simulink library "ESSLibrary"  (R2020a)
settings: Solver=VariableStepAuto  StartTime=0.0  StopTime=10.0  RelTol=1e-3
libraries: $bdroot x82, powerlib_meascontrol x10, simulink x7
(part 2 of 7)

== system ESSLibrary/PostProcessing ==
  Enable : Inport  OutDataTypeStr=boolean
  ECPAppPow : Inport  Port=2  OutDataTypeStr=double
  ActivePowerPU : Inport  Port=3  OutDataTypeStr=double
  ReactivePowerPU : Inport  Port=4  OutDataTypeStr=double
  ElseActionSubsystem : Subsystem  TreatAsAtomicUnit=on
  If : If  IfExpression=u1 ~= 0
  If Action Subsystem : Subsystem  TreatAsAtomicUnit=on
  Switch1 : Switch  Criteria=u2 > Threshold
  Switch28 : Switch  Criteria=u2 > Threshold
  ActivePowerOut : Outport
  ReactivePowerOut : Outport  Port=2
  wires:
  If/1 -> If Action Subsystem/Action
  If/2 -> ElseActionSubsystem/Action
  Enable/1 -> Switch28/2, Switch1/2, If/1
  ActivePowerPU/1 -> If Action Subsystem/2(ActivePowerPU)
  [ElseActivePowerOut] -> Switch28/3
  ECPAppPow/1 -> If Action Subsystem/1(ECPAppPow)
  ReactivePowerPU/1 -> If Action Subsystem/3(ReactivePowerPU)
  If Action Subsystem/2(ReactivePowerOut) -> [IfReactivePowerOut]
  If Action Subsystem/1(ActivePowerOut) -> [IfActivePowerOut]
  [IfActivePowerOut] -> Switch28/1
  [IfReactivePowerOut] -> Switch1/1
  [ElseReactivePowerOut] -> Switch1/3
  Switch28/1 -> ActivePowerOut/1
  Switch1/1 -> ReactivePowerOut/1
  ElseActionSubsystem/1(ActivePowerOut) -> [ElseActivePowerOut]
  ElseActionSubsystem/2(ReactivePowerOut) -> [ElseReactivePowerOut]

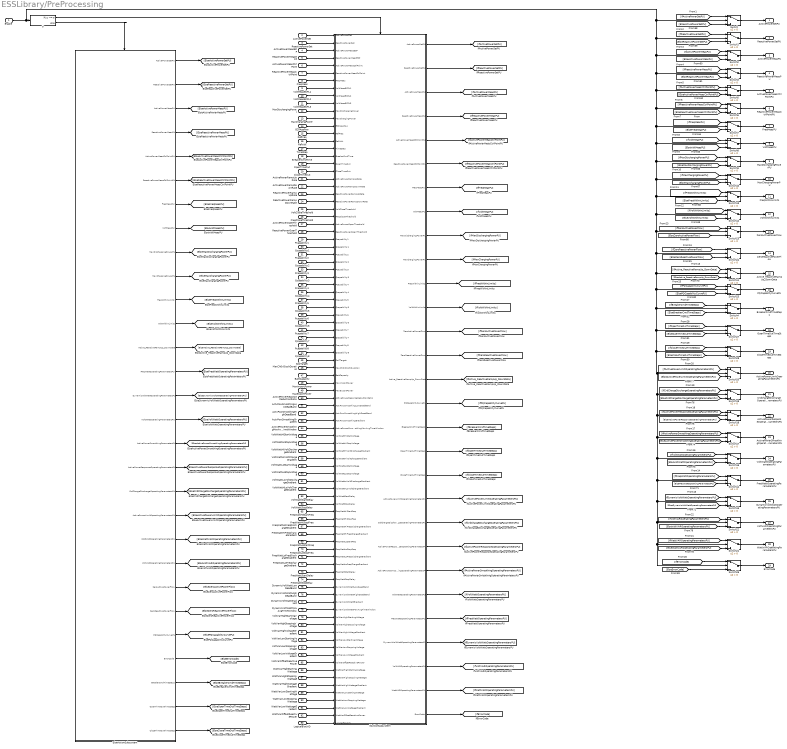
== system ESSLibrary/PreProcessing ==
  Enable : Inport  OutDataTypeStr=boolean
  ActivePowerSet : Inport  Port=2  OutDataTypeStr=double
  "ReactivePowerSet " : Inport  Port=3  OutDataTypeStr=double
  ActivePowerMeasECP : Inport  Port=4  OutDataTypeStr=double
  ReactivePowerMeasECP : Inport  Port=5  OutDataTypeStr=double
  ActivePowerMeasCtrlPoint : Inport  Port=6  OutDataTypeStr=double
  ReactivePowerMeasCtrlPoint : Inport  Port=7  OutDataTypeStr=double
  FreqMeas : Inport  Port=8  OutDataTypeStr=double
  VoltMeasECPL1 : Inport  Port=9  OutDataTypeStr=double
  VoltMeasECPL2 : Inport  Port=10  OutDataTypeStr=double
  VoltMeasECPL3 : Inport  Port=11  OutDataTypeStr=double
  MaxDischargingPower : Inport  Port=12  OutDataTypeStr=double
  MaxChargingPower : Inport  Port=13  OutDataTypeStr=double
  ECPAppPow : Inport  Port=14  OutDataTypeStr=double
  RefFreq : Inport  Port=15  OutDataTypeStr=double
  RefVolt : Inport  Port=16  OutDataTypeStr=double
  TimeStep : Inport  Port=17  OutDataTypeStr=double
  BreakerCmdTime : Inport  Port=18  OutDataTypeStr=double
  OpenTimeOut : Inport  Port=19  OutDataTypeStr=double
  CloseTimeOut : Inport  Port=20  OutDataTypeStr=double
  ActivePowerRampUpRate : Inport  Port=21  OutDataTypeStr=double
  ActivePowerRampDownRate : Inport  Port=22  OutDataTypeStr=double
  ReactivePowerRampUpRate : Inport  Port=23  OutDataTypeStr=double
  ReactivePowerRampDownRate : Inport  Port=24  OutDataTypeStr=double
  VoltCloseThreshold : Inport  Port=25  OutDataTypeStr=double
  FreqCloseThreshold : Inport  Port=26  OutDataTypeStr=double
  ActivePowerOpenThreshold : Inport  Port=27  OutDataTypeStr=double
  ReactivePowerOpenThreshold : Inport  Port=28  OutDataTypeStr=double
  Pcapability1 : Inport  Port=29  OutDataTypeStr=double
  Qcapability1 : Inport  Port=30  OutDataTypeStr=double
  Pcapability2 : Inport  Port=31  OutDataTypeStr=double
  Qcapability2 : Inport  Port=32  OutDataTypeStr=double
  Pcapability3 : Inport  Port=33  OutDataTypeStr=double
  Qcapability3 : Inport  Port=34  OutDataTypeStr=double
  Pcapability4 : Inport  Port=35  OutDataTypeStr=double
  Qcapability4 : Inport  Port=36  OutDataTypeStr=double
  Pcapability5 : Inport  Port=37  OutDataTypeStr=double
  Qcapability5 : Inport  Port=38  OutDataTypeStr=double
  Pcapability6 : Inport  Port=39  OutDataTypeStr=double
  Qcapability6 : Inport  Port=40  OutDataTypeStr=double
  Pcapability7 : Inport  Port=41  OutDataTypeStr=double
  Qcapability7 : Inport  Port=42  OutDataTypeStr=double
  Pcapability8 : Inport  Port=43  OutDataTypeStr=double
  Qcapability8 : Inport  Port=44  OutDataTypeStr=double
  SoCTarget : Inport  Port=45  OutDataTypeStr=double
  MaxChOrDischDuration : Inport  Port=46  OutDataTypeStr=double
  BattCapacity : Inport  Port=47  OutDataTypeStr=double
  MaxImportPower : Inport  Port=48  OutDataTypeStr=double
  MaxExportPower : Inport  Port=49  OutDataTypeStr=double
  ActivePowerReponseReductionRatio : Inport  Port=50  OutDataTypeStr=double
  ActvPowSmoothingLowDeadBand : Inport  Port=51  OutDataTypeStr=double
  ActvPowSmoothingHighDeadBand : Inport  Port=52  OutDataTypeStr=double
  ActvPowSmoothingGradient : Inport  Port=53  OutDataTypeStr=double
  ActivePowerSmoothingMovAvgTimeWindow : Inport  Port=54  OutDataTypeStr=double
  VoltWattHiStartVoltage : Inport  Port=55  OutDataTypeStr=double
  VoltWattHiStopVoltage : Inport  Port=56  OutDataTypeStr=double
  VoltWattHiVoltDischargeGradient : Inport  Port=57  OutDataTypeStr=double
  VoltWattHiVoltChargeGradient : Inport  Port=58  OutDataTypeStr=double
  VoltWattLoStartVoltage : Inport  Port=59  OutDataTypeStr=double
  VoltWattLoStopVoltage : Inport  Port=60  OutDataTypeStr=double
  VoltWattLoVoltDischargeGradient : Inport  Port=61  OutDataTypeStr=double
  VoltWattHLoVoltChargeGradient : Inport  Port=62  OutDataTypeStr=double
  VoltWattStartDelay : Inport  Port=63  OutDataTypeStr=double
  VoltWattStopDelay : Inport  Port=64  OutDataTypeStr=double
  FreqWattHiStartFreq : Inport  Port=65  OutDataTypeStr=double
  FreqWattHiStopFreq : Inport  Port=66  OutDataTypeStr=double
  FreqWattHiFreqDischargeGradient : Inport  Port=67  OutDataTypeStr=double
  FreqWattHiFreqChargeGradient : Inport  Port=68  OutDataTypeStr=double
  FreqWattLoStartFreq : Inport  Port=69  OutDataTypeStr=double
  FreqWattLoStopFreq : Inport  Port=70  OutDataTypeStr=double
  FreqWattLoFreqDischargeGradient : Inport  Port=71  OutDataTypeStr=double
  FreqWattLoFreqChargeGradient : Inport  Port=72  OutDataTypeStr=double
  FreqWattStartDelay : Inport  Port=73  OutDataTypeStr=double
  FreqWattStopDelay : Inport  Port=74  OutDataTypeStr=double
  DynamicVoltWattLowDeadBand : Inport  Port=75  OutDataTypeStr=double
  DynamicVoltWattHighDeadBand : Inport  Port=76  OutDataTypeStr=double
  DynamicVoltWattGradient : Inport  Port=77  OutDataTypeStr=double
  DynamicVoltWattMovAvgTimeWindow : Inport  Port=78  OutDataTypeStr=double
  VoltVarHighStartingVoltage : Inport  Port=79  OutDataTypeStr=double
  VoltVarHighStoppingVoltage : Inport  Port=80  OutDataTypeStr=double
  VoltVarHighVoltageGradient : Inport  Port=81  OutDataTypeStr=double
  VoltVarLowStartingVoltage : Inport  Port=82  OutDataTypeStr=double
  VoltVarLowStoppingVoltage : Inport  Port=83  OutDataTypeStr=double
  VoltVarLowVoltageGradient : Inport  Port=84  OutDataTypeStr=double
  VoltVarOffsetReactivePower : Inport  Port=85  OutDataTypeStr=double
  WattVarHighStartingWattage : Inport  Port=86  OutDataTypeStr=double
  WattVarHighStoppingWattage : Inport  Port=87  OutDataTypeStr=double
  WattVarHighWattageGradient : Inport  Port=88  OutDataTypeStr=double
  WattVarLowStartingWattage : Inport  Port=89  OutDataTypeStr=double
  WattVarLowStoppingWattage : Inport  Port=90  OutDataTypeStr=double
  WattVarLowWattageGradient : Inport  Port=91  OutDataTypeStr=double
  WattVarOffsetReactivePower : Inport  Port=92  OutDataTypeStr=double
  LogicalBlockID : Inport  Port=93  OutDataTypeStr=int32
  ElseActionSubsystem : Subsystem  TreatAsAtomicUnit=on
  If : If  IfExpression=u1 ~= 0
  IfActionSubsystem : Subsystem  TreatAsAtomicUnit=on
  Switch : Switch  Criteria=u2 > Threshold
  Switch{1..25,27..28} (27 alike) : Switch  Criteria=u2 > Threshold  OutDataTypeStr=Inherit: Inherit via back propagation
  Switch26 : Switch  Criteria=u2 > Threshold
  ActivePowerSetPU : Outport  OutDataTypeStr=double
  "ReactivePowerSetPU " : Outport  Port=2  OutDataTypeStr=double
  ActivePowerMeasPU : Outport  Port=3  OutDataTypeStr=double
  ReactivePowerMeasPU : Outport  Port=4  OutDataTypeStr=double
  ActivePowerMeasCtrlPointPU : Outport  Port=5  OutDataTypeStr=double
  ReactivePowerMeasCtrlPointPU : Outport  Port=6  OutDataTypeStr=double
  FreqMeasPU : Outport  Port=7  OutDataTypeStr=double
  VoltMeasPU : Outport  Port=8  OutDataTypeStr=double
  MaxDischargingPowerPU : Outport  Port=9  OutDataTypeStr=double
  MaxChargingPowerPU : Outport  Port=10  OutDataTypeStr=double
  FreqWithinLimits : Outport  Port=11  OutDataTypeStr=boolean
  VoltWithinLimits : Outport  Port=12  OutDataTypeStr=boolean
  ZeroActivePowerFlow : Outport  Port=13  OutDataTypeStr=boolean
  ZeroReactivePowerFlow : Outport  Port=14  OutDataTypeStr=boolean
  Active_ReactiveRampUp_DownData : Outport  Port=15  OutDataTypeStr=Bus: Active_ReactiveRampUp_DownData
  PQCapabiltyCurvePU : Outport  Port=16  OutDataTypeStr=double
  BreakerCmdTimeSteps : Outport  Port=17  OutDataTypeStr=int16
  OpenTimeOutTimeSteps : Outport  Port=18  OutDataTypeStr=int16
  CloseTimeOutTimeSteps : Outport  Port=19  OutDataTypeStr=int16
  ActivePowerLimitOperatingParametersPU : Outport  Port=20  OutDataTypeStr=Bus: ActivePowerLimitOperatingParametersPU
  CrdChargeDischargeOperatingParametersPU : Outport  Port=21
  ActivePowerResponseOperatingParametersPU : Outport  Port=22  OutDataTypeStr=Bus: ActivePowerResponseOperatingParametersPU
  ActivePowerSmoothingOperatingParametersPU : Outport  Port=23  OutDataTypeStr=Bus: ActivePowerSmoothingOperatingParametersPU
  VoltWattOperatingParametersPU : Outport  Port=24  OutDataTypeStr=Bus: VoltWattOperatingParametersPU
  FreqWattOperatingParametersPU : Outport  Port=25  OutDataTypeStr=Bus: FreqWattOperatingParametersPU
  DynamicVoltWattOperatingParametersPU : Outport  Port=26  OutDataTypeStr=Bus: DynamicVoltWattOperatingParameters
  VoltVAROperatingParametersPU : Outport  Port=27  OutDataTypeStr=Bus: VoltVarOperatingParametersPU
  WattVAROperatingParametersPU : Outport  Port=28  OutDataTypeStr=Bus: WattVarOperatingParametersPU
  ErrorCode : Outport  Port=29  OutDataTypeStr=uint32
  wires:
  If/1 -> IfActionSubsystem/Action
  If/2 -> ElseActionSubsystem/Action
  ActivePowerSet/1 -> IfActionSubsystem/1(ActivePowerSet)
  MaxDischargingPower/1 -> IfActionSubsystem/11(MaxDischargingPower)
  MaxChargingPower/1 -> IfActionSubsystem/12(MaxChargingPower)
  "ReactivePowerSet "/1 -> IfActionSubsystem/2("ReactivePowerSet ")
  ActivePowerMeasECP/1 -> IfActionSubsystem/3(ActivePowerMeasECP)
  ReactivePowerMeasECP/1 -> IfActionSubsystem/4(ReactivePowerMeasECP)
  ActivePowerMeasCtrlPoint/1 -> IfActionSubsystem/5(ActivePowerMeasCtrlPoint)
  ReactivePowerMeasCtrlPoint/1 -> IfActionSubsystem/6(ReactivePowerMeasCtrlPoint)
  ActivePowerOpenThreshold/1 -> IfActionSubsystem/26(ActivePowerOpenThreshold)
  FreqMeas/1 -> IfActionSubsystem/7(FreqMeas)
  FreqCloseThreshold/1 -> IfActionSubsystem/25(FreqCloseThreshold)
  VoltMeasECPL1/1 -> IfActionSubsystem/8(VoltMeasECPL1)
  VoltMeasECPL2/1 -> IfActionSubsystem/9(VoltMeasECPL2)
  VoltMeasECPL3/1 -> IfActionSubsystem/10(VoltMeasECPL3)
  RefVolt/1 -> IfActionSubsystem/15(RefVolt)
  RefFreq/1 -> IfActionSubsystem/14(RefFreq)
  ECPAppPow/1 -> IfActionSubsystem/13(ECPAppPow)
  VoltCloseThreshold/1 -> IfActionSubsystem/24(VoltCloseThreshold)
  ReactivePowerOpenThreshold/1 -> IfActionSubsystem/27(ReactivePowerOpenThreshold)
  IfActionSubsystem/29(ErrorCode) -> [IfErrorCode]
  IfActionSubsystem/8(VoltMeasPU) -> [IfVoltMeasPU]
  IfActionSubsystem/7(FreqMeasPU) -> [IfFreqMeasPU]
  IfActionSubsystem/6(ReactivePowerMeasCtrlPointPU) -> [IfReactivePowerMeasCtrlPointPU]
  IfActionSubsystem/5(ActivePowerMeasCtrlPointPU) -> [IfActivePowerMeasCtrlPointPU]
  IfActionSubsystem/4(ReactivePowerMeasPU) -> [IfReactivePowerMeasPU]
  IfActionSubsystem/2("ReactivePowerSetPU ") -> [IfReactivePowerSetPU]
  IfActionSubsystem/3(ActivePowerMeasPU) -> [IfActivePowerMeasPU]
  IfActionSubsystem/1(ActivePowerSetPU) -> [IfActivePowerSetPU]
  IfActionSubsystem/9(MaxDischargingPowerPU) -> [IfMaxDischargingPowerPU]
  IfActionSubsystem/10(MaxChargingPowerPU) -> [IfMaxChargingPowerPU]
  Switch/1 -> ActivePowerSetPU/1
  Switch1/1 -> "ReactivePowerSetPU "/1
  Switch2/1 -> ActivePowerMeasPU/1
  Switch3/1 -> ReactivePowerMeasPU/1
  Switch5/1 -> ActivePowerMeasCtrlPointPU/1
  Switch6/1 -> ReactivePowerMeasCtrlPointPU/1
  Switch7/1 -> FreqMeasPU/1
  Switch8/1 -> VoltMeasPU/1
  Switch9/1 -> MaxDischargingPowerPU/1
  Switch10/1 -> MaxChargingPowerPU/1
  IfActionSubsystem/11(FreqWithinLimits) -> [IfFreqWithinLimits]
  IfActionSubsystem/12(VoltWithinLimits) -> [IfVoltWithinLimits]
  Switch12/1 -> VoltWithinLimits/1
  Switch13/1 -> FreqWithinLimits/1
  Enable/1 -> Switch/2, Switch1/2, Switch2/2, Switch3/2, Switch5/2, Switch6/2, Switch7/2, Switch8/2, Switch9/2, Switch10/2, Switch13/2, Switch12/2, Switch23/2, Switch11/2, Switch4/2, Switch28/2, Switch20/2, Switch26/2, Switch21/2, Switch22/2, Switch15/2, Switch14/2, Switch16/2, Switch17/2, Switch18/2, Switch19/2, Switch27/2, Switch25/2, Switch24/2, If/1
  ReactivePowerRampUpRate/1 -> IfActionSubsystem/22(ReactivePowerRampUpRate)
  ReactivePowerRampDownRate/1 -> IfActionSubsystem/23(ReactivePowerRampDownRate)
  ActivePowerRampDownRate/1 -> IfActionSubsystem/21(ActivePowerRampDownRate)
  ActivePowerRampUpRate/1 -> IfActionSubsystem/20(ActivePowerRampUpRate)
  TimeStep/1 -> IfActionSubsystem/16(TimeStep)
  MaxImportPower/1 -> IfActionSubsystem/47(MaxImportPower)
  WattVarLowStartingWattage/1 -> IfActionSubsystem/88(WattVarLowStartingWattage)
  WattVarHighWattageGradient/1 -> IfActionSubsystem/87(WattVarHighWattageGradient)
  FreqWattHiStartFreq/1 -> IfActionSubsystem/64(FreqWattHiStartFreq)
  FreqWattHiStopFreq/1 -> IfActionSubsystem/65(FreqWattHiStopFreq)
  FreqWattHiFreqDischargeGradient/1 -> IfActionSubsystem/66(FreqWattHiFreqDischargeGradient)
  FreqWattHiFreqChargeGradient/1 -> IfActionSubsystem/67(FreqWattHiFreqChargeGradient)
  FreqWattLoStopFreq/1 -> IfActionSubsystem/69(FreqWattLoStopFreq)
  FreqWattLoStartFreq/1 -> IfActionSubsystem/68(FreqWattLoStartFreq)
  FreqWattLoFreqDischargeGradient/1 -> IfActionSubsystem/70(FreqWattLoFreqDischargeGradient)
  FreqWattLoFreqChargeGradient/1 -> IfActionSubsystem/71(FreqWattLoFreqChargeGradient)
  DynamicVoltWattHighDeadBand/1 -> IfActionSubsystem/75(DynamicVoltWattHighDeadBand)
  DynamicVoltWattLowDeadBand/1 -> IfActionSubsystem/74(DynamicVoltWattLowDeadBand)
  DynamicVoltWattGradient/1 -> IfActionSubsystem/76(DynamicVoltWattGradient)
  DynamicVoltWattMovAvgTimeWindow/1 -> IfActionSubsystem/77(DynamicVoltWattMovAvgTimeWindow)
  VoltWattHiStartVoltage/1 -> IfActionSubsystem/54(VoltWattHiStartVoltage)
  VoltWattHiStopVoltage/1 -> IfActionSubsystem/55(VoltWattHiStopVoltage)
  VoltWattHiVoltDischargeGradient/1 -> IfActionSubsystem/56(VoltWattHiVoltDischargeGradient)
  VoltWattHiVoltChargeGradient/1 -> IfActionSubsystem/57(VoltWattHiVoltChargeGradient)
  ActvPowSmoothingLowDeadBand/1 -> IfActionSubsystem/50(ActvPowSmoothingLowDeadBand)
  ActvPowSmoothingHighDeadBand/1 -> IfActionSubsystem/51(ActvPowSmoothingHighDeadBand)
  ActivePowerSmoothingMovAvgTimeWindow/1 -> IfActionSubsystem/53(ActivePowerSmoothingMovAvgTimeWindow)
  ActivePowerReponseReductionRatio/1 -> IfActionSubsystem/49(ActivePowerReponseReductionRatio)
  SoCTarget/1 -> IfActionSubsystem/44(SoCTarget)
  MaxChOrDischDuration/1 -> IfActionSubsystem/45(MaxChOrDischDuration)
  WattVarHighStartingWattage/1 -> IfActionSubsystem/85(WattVarHighStartingWattage)
  WattVarHighStoppingWattage/1 -> IfActionSubsystem/86(WattVarHighStoppingWattage)
  VoltVarHighStartingVoltage/1 -> IfActionSubsystem/78(VoltVarHighStartingVoltage)
  VoltVarHighStoppingVoltage/1 -> IfActionSubsystem/79(VoltVarHighStoppingVoltage)
  VoltVarHighVoltageGradient/1 -> IfActionSubsystem/80(VoltVarHighVoltageGradient)
  VoltVarLowStartingVoltage/1 -> IfActionSubsystem/81(VoltVarLowStartingVoltage)
  Pcapability1/1 -> IfActionSubsystem/28(Pcapability1)
  Qcapability1/1 -> IfActionSubsystem/29(Qcapability1)
  Pcapability2/1 -> IfActionSubsystem/30(Pcapability2)
  Qcapability2/1 -> IfActionSubsystem/31(Qcapability2)
  Pcapability3/1 -> IfActionSubsystem/32(Pcapability3)
  Qcapability3/1 -> IfActionSubsystem/33(Qcapability3)
  Pcapability4/1 -> IfActionSubsystem/34(Pcapability4)
  Qcapability4/1 -> IfActionSubsystem/35(Qcapability4)
  Pcapability5/1 -> IfActionSubsystem/36(Pcapability5)
  Qcapability5/1 -> IfActionSubsystem/37(Qcapability5)
  Pcapability6/1 -> IfActionSubsystem/38(Pcapability6)
  Qcapability6/1 -> IfActionSubsystem/39(Qcapability6)
  Pcapability7/1 -> IfActionSubsystem/40(Pcapability7)
  Qcapability7/1 -> IfActionSubsystem/41(Qcapability7)
  Pcapability8/1 -> IfActionSubsystem/42(Pcapability8)
  Qcapability8/1 -> IfActionSubsystem/43(Qcapability8)
  LogicalBlockID/1 -> IfActionSubsystem/92(LogicalBlockID)
  ActvPowSmoothingGradient/1 -> IfActionSubsystem/52(ActvPowSmoothingGradient)
  WattVarLowWattageGradient/1 -> IfActionSubsystem/90(WattVarLowWattageGradient)
  VoltVarOffsetReactivePower/1 -> IfActionSubsystem/84(VoltVarOffsetReactivePower)
  VoltVarLowVoltageGradient/1 -> IfActionSubsystem/83(VoltVarLowVoltageGradient)
  VoltVarLowStoppingVoltage/1 -> IfActionSubsystem/82(VoltVarLowStoppingVoltage)
  BattCapacity/1 -> IfActionSubsystem/46(BattCapacity)
  MaxExportPower/1 -> IfActionSubsystem/48(MaxExportPower)
  VoltWattLoStartVoltage/1 -> IfActionSubsystem/58(VoltWattLoStartVoltage)
  VoltWattLoStopVoltage/1 -> IfActionSubsystem/59(VoltWattLoStopVoltage)
  VoltWattLoVoltDischargeGradient/1 -> IfActionSubsystem/60(VoltWattLoVoltDischargeGradient)
  VoltWattHLoVoltChargeGradient/1 -> IfActionSubsystem/61(VoltWattHLoVoltChargeGradient)
  VoltWattStartDelay/1 -> IfActionSubsystem/62(VoltWattStartDelay)
  VoltWattStopDelay/1 -> IfActionSubsystem/63(VoltWattStopDelay)
  WattVarLowStoppingWattage/1 -> IfActionSubsystem/89(WattVarLowStoppingWattage)
  WattVarOffsetReactivePower/1 -> IfActionSubsystem/91(WattVarOffsetReactivePower)
  FreqWattStopDelay/1 -> IfActionSubsystem/73(FreqWattStopDelay)
  FreqWattStartDelay/1 -> IfActionSubsystem/72(FreqWattStartDelay)
  IfActionSubsystem/15(Active_ReactiveRampUp_DownData) -> [IfActive_ReactiveRampUp_DownData]
  IfActionSubsystem/25(FreqWattOperatingParametersPU) -> [IfFreqWattOperatingParametersPU]
  IfActionSubsystem/26(DynamicVoltWattOperatingParametersPU) -> [IfDynamicVoltWattOperatingParametersPU]
  IfActionSubsystem/24(VoltWattOperatingParametersPU) -> [IfVoltWattOperatingParametersPU]
  IfActionSubsystem/23(ActivePowerSmoothingOperatingParametersPU) -> [IfActivePowerSmoothingOperatingParametersPU]
  IfActionSubsystem/21(CrdChargeDischargeOperatingParametersPU) -> [IfCrdChargeDischargeOperatingParametersPU]
  IfActionSubsystem/20(ActivePowerLimitOperatingParametersPU) -> [IfActivePowerLimitOperatingParametersPU]
  IfActionSubsystem/28(WattVAROperatingParametersPU) -> [IfWattVAROperatingParametersPU]
  IfActionSubsystem/27(VoltVAROperatingParametersPU) -> [IfVoltVAROperatingParametersPU]
  IfActionSubsystem/13(ZeroActivePowerFlow) -> [IfZeroActivePowerFlow]
  IfActionSubsystem/14(ZeroReactivePowerFlow) -> [IfZeroReactivePowerFlow]
  IfActionSubsystem/16(PQCapabiltyCurvePU) -> [IfPQCapabilityCurvePU]
  ElseActionSubsystem/1(ActivePowerSetPU) -> [ElseActivePowerSetPU]
  ElseActionSubsystem/2("ReactivePowerSetPU ") -> [ElseReactivePowerSetPU]
  ElseActionSubsystem/3(ActivePowerMeasPU) -> [ElseActivePowerMeasPU]
  ElseActionSubsystem/4(ReactivePowerMeasPU) -> [ElseReactivePowerMeasPU]
  ElseActionSubsystem/5(ActivePowerMeasCtrlPointPU) -> [ElseActivePowerMeasCtrlPointPU]
  ElseActionSubsystem/6(ReactivePowerMeasCtrlPointPU) -> [ElseReactivePowerMeasCtrlPointPU]
  ElseActionSubsystem/7(FreqMeasPU) -> [ElseFreqMeasPU]
  ElseActionSubsystem/8(VoltMeasPU) -> [ElseVoltMeasPU]
  ElseActionSubsystem/9(MaxDischargingPowerPU) -> [ElseMaxDischargingPowerPU]
  ElseActionSubsystem/10(MaxChargingPowerPU) -> [ElseMaxChargingPowerPU]
  ElseActionSubsystem/11(FreqWithinLimits) -> [ElseFreqWithinLimits]
  ElseActionSubsystem/12(VoltWithinLimits) -> [ElseVoltWithinLimits]
  ElseActionSubsystem/13(Active_ReactiveRampUp_DownData) -> [ElseActive_ReactiveRampUp_DownData]
  ElseActionSubsystem/14(FreqWattOperatingParametersPU) -> [ElseFreqWattOperatingParametersPU]
  ElseActionSubsystem/15(DynamicVoltWattOperatingParametersPU) -> [ElseDynamicVoltWattOperatingParametersPU]
  ElseActionSubsystem/16(VoltWattOperatingParametersPU) -> [ElseVoltWattOperatingParametersPU]
  ElseActionSubsystem/17(ActivePowerSmoothingParametersPU) -> [ElseActivePowerSmoothingOperatingParametersPU]
  ElseActionSubsystem/18(ActivePowerResponseOperatingParametersPU) -> [ElseActivePowerResponseOperatingParametersPU]
  ElseActionSubsystem/19(CrdChargeDischargeOperatingParametersPU) -> [ElseCrdChargeDischargeOperatingParametersPU]
  ElseActionSubsystem/20(ActivePowerLimitOperatingParametersPU) -> [ElseActivePowerLimitOperatingParametersPU]
  ElseActionSubsystem/21(WattVAROperatingParametersPU) -> [ElseWattVAROperatingParametersPU]
  ElseActionSubsystem/22(VoltVAROperatingParametersPU) -> [ElseVoltVAROperatingParametersPU]
  ElseActionSubsystem/23(ZeroActivePowerFlow) -> [ElseZeroActivePowerFlow]
  ElseActionSubsystem/24(ZeroReactivePowerFlow) -> [ElseZeroReactivePowerFlow]
  ElseActionSubsystem/25(PQCapabiltyCurvePU) -> [ElsePQCapabilityCurvePU]
  ElseActionSubsystem/26(ErrorCode) -> [ElseErrorCode]
  [ElseActivePowerSetPU] -> Switch/3
  [ElseReactivePowerSetPU] -> Switch1/3
  [ElseActivePowerMeasPU] -> Switch2/3
  [ElseReactivePowerMeasPU] -> Switch3/3
  [ElseActivePowerMeasCtrlPointPU] -> Switch5/3
  [ElseReactivePowerMeasCtrlPointPU] -> Switch6/3
  [ElseFreqMeasPU] -> Switch7/3
  [ElseVoltMeasPU] -> Switch8/3
  [ElseMaxDischargingPowerPU] -> Switch9/3
  [ElseMaxChargingPowerPU] -> Switch10/3
  [ElseFreqWithinLimits] -> Switch13/3
  [ElseVoltWithinLimits] -> Switch12/3
  [ElseActive_ReactiveRampUp_DownData] -> Switch11/3
  [ElseFreqWattOperatingParametersPU] -> Switch14/3
  [ElseDynamicVoltWattOperatingParametersPU] -> Switch15/3
  [ElseVoltWattOperatingParametersPU] -> Switch16/3
  [ElseActivePowerSmoothingOperatingParametersPU] -> Switch17/3
  [ElseActivePowerResponseOperatingParametersPU] -> Switch18/3
  [ElseCrdChargeDischargeOperatingParametersPU] -> Switch19/3
  [ElseActivePowerLimitOperatingParametersPU] -> Switch20/3
  [ElseWattVAROperatingParametersPU] -> Switch21/3
  [ElseVoltVAROperatingParametersPU] -> Switch22/3
  [ElseZeroActivePowerFlow] -> Switch23/3
  [ElseZeroReactivePowerFlow] -> Switch24/3
  [ElsePQCapabilityCurvePU] -> Switch25/3
  [ElseErrorCode] -> Switch26/3
  [IfActivePowerSetPU] -> Switch/1
  [IfReactivePowerSetPU] -> Switch1/1
  [IfActivePowerMeasPU] -> Switch2/1
  [IfReactivePowerMeasPU] -> Switch3/1
  [IfActivePowerMeasCtrlPointPU] -> Switch5/1
  [IfReactivePowerMeasCtrlPointPU] -> Switch6/1
  [IfFreqMeasPU] -> Switch7/1
  [IfVoltMeasPU] -> Switch8/1
  [IfMaxDischargingPowerPU] -> Switch9/1
  [IfMaxChargingPowerPU] -> Switch10/1
  [IfFreqWithinLimits] -> Switch13/1
  [IfVoltWithinLimits] -> Switch12/1
  [IfActive_ReactiveRampUp_DownData] -> Switch11/1
  [IfFreqWattOperatingParametersPU] -> Switch14/1
  [IfDynamicVoltWattOperatingParametersPU] -> Switch15/1
  [IfVoltWattOperatingParametersPU] -> Switch16/1
  [IfActivePowerSmoothingOperatingParametersPU] -> Switch17/1
  [IfActivePowerResponseOperatingParametersPU] -> Switch18/1
  [IfCrdChargeDischargeOperatingParametersPU] -> Switch19/1
  [IfActivePowerLimitOperatingParametersPU] -> Switch20/1
  [IfWattVAROperatingParametersPU] -> Switch21/1
  [IfVoltVAROperatingParametersPU] -> Switch22/1
  [IfZeroActivePowerFlow] -> Switch23/1
  [IfZeroReactivePowerFlow] -> Switch24/1
  [IfPQCapabilityCurvePU] -> Switch25/1
  [IfErrorCode] -> Switch26/1
  IfActionSubsystem/22(ActivePowerResponseOperatingParametersPU) -> [IfActivePowerResponseOperatingParametersPU]
  Switch14/1 -> FreqWattOperatingParametersPU/1
  Switch15/1 -> DynamicVoltWattOperatingParametersPU/1
  Switch16/1 -> VoltWattOperatingParametersPU/1
  Switch17/1 -> ActivePowerSmoothingOperatingParametersPU/1
  Switch18/1 -> ActivePowerResponseOperatingParametersPU/1
  Switch19/1 -> CrdChargeDischargeOperatingParametersPU/1
  Switch20/1 -> ActivePowerLimitOperatingParametersPU/1
  Switch21/1 -> WattVAROperatingParametersPU/1
  Switch22/1 -> VoltVAROperatingParametersPU/1
  Switch23/1 -> ZeroActivePowerFlow/1
  Switch24/1 -> ZeroReactivePowerFlow/1
  Switch25/1 -> PQCapabiltyCurvePU/1
  Switch26/1 -> ErrorCode/1
  BreakerCmdTime/1 -> IfActionSubsystem/17(BreakerCmdTime)
  OpenTimeOut/1 -> IfActionSubsystem/18(OpenTimeOut)
  CloseTimeOut/1 -> IfActionSubsystem/19(CloseTimeOut)
  IfActionSubsystem/17(BreakerCmdTimeSteps) -> [IfBreakerCmdTimeSteps]
  IfActionSubsystem/18(OpenTimeOutTimeSteps) -> [IfOpenTimeOutTimeSteps]
  IfActionSubsystem/19(CloseTimeOutTimeSteps) -> [IfCloseTimeOutTimeSteps]
  ElseActionSubsystem/27(BreakerCmdTimeSteps) -> [ElseBreakerCmdTimeSteps]
  ElseActionSubsystem/28(OpenTimeOutTimeSteps) -> [ElseOpenTimeOutTimeSteps]
  ElseActionSubsystem/29(CloseTimeOutTimeSteps) -> [ElseCloseTimeOutTimeSteps]
  Switch28/1 -> CloseTimeOutTimeSteps/1
  Switch27/1 -> OpenTimeOutTimeSteps/1
  Switch4/1 -> BreakerCmdTimeSteps/1
  [IfBreakerCmdTimeSteps] -> Switch4/1
  [IfOpenTimeOutTimeSteps] -> Switch27/1
  [IfCloseTimeOutTimeSteps] -> Switch28/1
  [ElseCloseTimeOutTimeSteps] -> Switch28/3
  [ElseOpenTimeOutTimeSteps] -> Switch27/3
  [ElseBreakerCmdTimeSteps] -> Switch4/3
  Switch11/1 -> Active_ReactiveRampUp_DownData/1

== system ESSLibrary/QReference_PF ==
  EnableDisable : Inport
  PFSet : Inport  Port=2
  PFSign : Inport  Port=3
  PSet : Inport  Port=4
  Enable1 : InportShadow
  If : If  IfExpression=u1 ~= 0
  If Action Subsystem : Subsystem  TreatAsAtomicUnit=on
  If Action Subsystem1 : Subsystem  TreatAsAtomicUnit=on
  Switch : Switch  Criteria=u2 > Threshold
  Switch1 : Switch  Criteria=u2 > Threshold
  PFSetQOut : Outport
  ErrorCode : Outport  Port=2
  wires:
  [ElsePFSetQSetPU] -> Switch1/3
  [IfPFSetQSetPU] -> Switch1/1
  [IfErrorCode] -> Switch/1
  [ElseErrorCode] -> Switch/3
  If Action Subsystem/2(ErrorCode) -> [IfErrorCode]
  If Action Subsystem1/2(ErrorCode) -> [ElseErrorCode]
  Enable1/1 -> Switch/2, Switch1/2
  Switch1/1 -> PFSetQOut/1
  Switch/1 -> ErrorCode/1
  PSet/1 -> If Action Subsystem/3(PSet)
  PFSet/1 -> If Action Subsystem/1(PFSet)
  If/2 -> If Action Subsystem1/Action
  If/1 -> If Action Subsystem/Action
  EnableDisable/1 -> If/1
  PFSign/1 -> If Action Subsystem/2(PFSign)
  If Action Subsystem/1(PFSetQSet) -> [IfPFSetQSetPU]
  If Action Subsystem1/1(PFSetQSetPU) -> [ElsePFSetQSetPU]

== system ESSLibrary/SaturationLimits ==
  InSignal : Inport
  UpperLimit : Inport  Port=2  OutDataTypeStr=double
  LowerLimit : Inport  Port=3  OutDataTypeStr=double
  GT : RelationalOperator  Operator=>  OutDataTypeStr=boolean  RndMeth=Simplest
  LT : RelationalOperator  Operator=<  OutDataTypeStr=boolean  RndMeth=Simplest
  Switch2 : Switch  Criteria=u2 > Threshold
  Switch3 : Switch  Criteria=u2 > Threshold
  OutSignal : Outport
  wires:
  Switch2/1 -> Switch3/1, LT/1
  UpperLimit/1 -> Switch2/3, GT/2
  LowerLimit/1 -> Switch3/3, LT/2
  GT/1 -> Switch2/2
  Switch3/1 -> OutSignal/1
  LT/1 -> Switch3/2
  InSignal/1 -> Switch2/1, GT/1

== system ESSLibrary/SoCManagement ==
  Enable : Inport  OutDataTypeStr=boolean
  ActivePowerMeasECP : Inport  Port=2  OutDataTypeStr=double
  SoCMeas : Inport  Port=3  OutDataTypeStr=double
  SoCMin : Inport  Port=4  OutDataTypeStr=double
  SoCMax : Inport  Port=5  OutDataTypeStr=double
  BattCapacity : Inport  Port=6  OutDataTypeStr=double
  ECPAppPow : Inport  Port=7  OutDataTypeStr=double
  TimeStep : Inport  Port=8  OutDataTypeStr=double
  ActiveReactivePowerRampUpDownData : Inport  Port=9  OutDataTypeStr=double
  LogicalBlockID : Inport  Port=10  OutDataTypeStr=int64
  ElseActionSubsystem : Subsystem  TreatAsAtomicUnit=on
  If : If  IfExpression=u1 ~= 0
  IfActionSubsystem : Subsystem  TreatAsAtomicUnit=on
  Switch{2..6} (5 alike) : Switch  Criteria=u2 > Threshold
  SoCFinal : Outport
  SoCNextStep : Outport  Port=2
  ChargeEnable : Outport  Port=3
  DischargeEnable : Outport  Port=4
  ErrorCode : Outport  Port=5  OutDataTypeStr=int64
  wires:
  Switch4/1 -> ErrorCode/1
  If/2 -> ElseActionSubsystem/Action
  If/1 -> IfActionSubsystem/Action
  ElseActionSubsystem/3(ChargeEnable) -> [ElseChargeEnable]
  ElseActionSubsystem/4(DischargeEnable) -> [ElseDischargeEnable]
  [ElseErrorCode] -> Switch4/3
  [ElseChargeEnable] -> Switch2/3
  [IfChargeEnable] -> Switch2/1
  [IfDischargeEnable] -> Switch3/1
  [ElseDischargeEnable] -> Switch3/3
  [IfErrorCode] -> Switch4/1
  Switch2/1 -> ChargeEnable/1
  Switch3/1 -> DischargeEnable/1
  IfActionSubsystem/4(DischargeEnable) -> [IfDischargeEnable]
  IfActionSubsystem/3(ChargeEnable) -> [IfChargeEnable]
  ElseActionSubsystem/5(ErrorCodeOut) -> [ElseErrorCode]
  ElseActionSubsystem/1(SoCFinal) -> [ElseSoCFinal]
  IfActionSubsystem/1(SoCFinal) -> [IfSoCFinal]
  Switch5/1 -> SoCFinal/1
  Enable/1 -> Switch5/2, Switch6/2, Switch4/2, Switch3/2, Switch2/2, If/1
  [IfSoCFinal] -> Switch5/1
  [ElseSoCFinal] -> Switch5/3
  IfActionSubsystem/2(SoCNextStep) -> [IfSoCNextStep]
  ElseActionSubsystem/2(SoCNextStep) -> [ElseSoCNextStep]
  Switch6/1 -> SoCNextStep/1
  [ElseSoCNextStep] -> Switch6/3
  [IfSoCNextStep] -> Switch6/1
  IfActionSubsystem/5(ErrorCodeOut) -> [IfErrorCode]
  ActivePowerMeasECP/1 -> IfActionSubsystem/1(ActivePowerMeasECP)
  SoCMeas/1 -> IfActionSubsystem/2(SoCMeas)
  SoCMin/1 -> IfActionSubsystem/3(SoCMin)
  SoCMax/1 -> IfActionSubsystem/4(SoCMax)
  BattCapacity/1 -> IfActionSubsystem/5(BattCapacity)
  ECPAppPow/1 -> IfActionSubsystem/6(ECPAppPow)
  TimeStep/1 -> IfActionSubsystem/7(TimeStep)
  LogicalBlockID/1 -> IfActionSubsystem/9(LogicalBlockID)
  ActiveReactivePowerRampUpDownData/1 -> IfActionSubsystem/8(ActiveReactivePowerRampUpDownData)

== system ESSLibrary/VoltVarMode ==
  VoltMeasPU : Inport
  VoltVarOperatingParametersPU : Inport  Port=2  OutDataTypeStr=Bus: VoltVarOperatingParametersPU
  Action Port : ActionPort
  Bus Selector2 : BusSelector  OutputSignals=VoltVarHighStartingVoltagePU,VoltVarHighStoppingVoltagePU,VoltVarHighVoltageGradientPU,VoltVarLowStartingVoltagePU,VoltVarLowStoppingVoltagePU,VoltVarLowVoltageGradientPU,VoltVarOffsetReactivePowerPU
  Constant1 : Constant  Value=0.0  OutDataTypeStr=double  SampleTime=-1
  TwoQuadrantDroop_PointBased : MATLAB Function  TreatAsAtomicUnit=on
  ReactivePowerOut : Outport  OutDataTypeStr=double
  wires:
  VoltVarOperatingParametersPU/1 -> Bus Selector2/1
  TwoQuadrantDroop_PointBased/1(Y_Out) -> ReactivePowerOut/1
  VoltMeasPU/1 -> TwoQuadrantDroop_PointBased/1(X_In)
  Constant1/1 -> TwoQuadrantDroop_PointBased/10(StopDelay), TwoQuadrantDroop_PointBased/9(StartDelay)
  Bus Selector2/4 -> TwoQuadrantDroop_PointBased/5(X_Lo_Stop)  "<VoltVarLowStartingVoltagePU>"
  Bus Selector2/3 -> TwoQuadrantDroop_PointBased/4(X_Lo_Start)  "<VoltVarHighVoltageGradientPU>"
  Bus Selector2/5 -> TwoQuadrantDroop_PointBased/6(X_Hi_Gradient)  "<VoltVarLowStoppingVoltagePU>"
  Bus Selector2/2 -> TwoQuadrantDroop_PointBased/3(X_Hi_Stop)  "<VoltVarHighStoppingVoltagePU>"
  Bus Selector2/6 -> TwoQuadrantDroop_PointBased/7(X_Lo_Gradient)  "<VoltVarLowVoltageGradientPU>"
  Bus Selector2/1 -> TwoQuadrantDroop_PointBased/2(X_Hi_Start)  "<VoltVarHighStartingVoltagePU>"
  Bus Selector2/7 -> TwoQuadrantDroop_PointBased/8(Y_Offset)  "<VoltVarOffsetReactivePowerPU>"

== system ESSLibrary/VoltWattMode ==
  VoltMeasPU : Inport
  ActivePowerMeasPU : Inport  Port=2
  VoltWattOperatingParametersPU : Inport  Port=3  OutDataTypeStr=Bus: VoltWattOperatingParametersPU
  MaxDischargingPowerPU : Inport  Port=4  OutDataTypeStr=double
  MaxChargingPowerPU : Inport  Port=5  OutDataTypeStr=double
  LogicalBlockID : Inport  Port=6  OutDataTypeStr=int64
  Action Port : ActionPort
  Bus Selector4 : BusSelector  OutputSignals=VoltWattHiStartVoltagePU,VoltWattHiStopVoltagePU,VoltWattHiDischargeGradientPU,VoltWattHiChargeGradientPU,VoltWattLoStartVoltagePU,VoltWattLoStopVoltagePU,VoltWattLoDischargeGradientPU,VoltWattLoChargeGradientPU,VoltWattStartDelay,VoltWattStopDelay
  Comparator : $bdroot/ChargeDischargeStorageMode/Comparator  SystemSampleTime=-1  Latency=0  AutoFrameSizeCalculation=off
  Constant10 : Constant  Value=0  OutDataTypeStr=int64
  Constant11 : Constant  Value=0  OutDataTypeStr=int64
  Constant2 : Constant  Value=2  OutDataTypeStr=int32
  Constant3 : Constant  Value=0  OutDataTypeStr=int8
  Constant5 : Constant  Value=0  OutDataTypeStr=int8
  Constant6 : Constant  OutDataTypeStr=boolean
  Equal2 : RelationalOperator  Operator=>  OutDataTypeStr=boolean  RndMeth=Simplest
  Gain1 : Gain  Gain=1000000
  MATLAB Function : MATLAB Function  TreatAsAtomicUnit=on
  MaxChargingPowerPU1 : InportShadow  Port=5  OutDataTypeStr=double
  MaxDischargingPowerPU1 : InportShadow  Port=4  OutDataTypeStr=double
  SaturationLimits : $bdroot/SaturationLimits  SystemSampleTime=-1  Latency=0  AutoFrameSizeCalculation=off
  Sum2 : Sum  OutDataTypeStr=int64
  Switch4 : Switch  Criteria=u2 > Threshold
  Terminator : Terminator
  Terminator1 : Terminator
  VariableIdentifier : Constant  OutDataTypeStr=int64
  ActivePowerOut : Outport
  ErrorCode : Outport  Port=2  OutDataTypeStr=int64
  wires:
  VoltWattOperatingParametersPU/1 -> Bus Selector4/1
  VoltMeasPU/1 -> MATLAB Function/1(X_In)
  ActivePowerMeasPU/1 -> MATLAB Function/2(Y_In)
  MaxDischargingPowerPU/1 -> SaturationLimits/2
  MATLAB Function/1(Y_Out) -> SaturationLimits/1, Comparator/2
  Sum2/1 -> Switch4/1
  Constant10/1 -> Equal2/2
  Comparator/3 -> Terminator1/1
  Constant2/1 -> Comparator/5
  Constant5/1 -> Comparator/7
  LogicalBlockID/1 -> Gain1/1
  VariableIdentifier/1 -> Comparator/8
  Constant6/1 -> Comparator/1
  Switch4/1 -> ErrorCode/1
  Constant11/1 -> Switch4/3
  Comparator/2 -> Terminator/1
  Comparator/1 -> Equal2/1, Sum2/1
  Gain1/1 -> Sum2/2
  Constant3/1 -> Comparator/6
  MaxDischargingPowerPU1/1 -> Comparator/3
  MaxChargingPowerPU/1 -> SaturationLimits/3
  Equal2/1 -> Switch4/2
  MaxChargingPowerPU1/1 -> Comparator/4
  SaturationLimits/1 -> ActivePowerOut/1
  [VoltWattHiStartVoltagePU] -> MATLAB Function/3(HiStartX)
  [VoltWattHiStopVoltagePU] -> MATLAB Function/4(HiStopX)
  [VoltWattHiDischargeGradientPU] -> MATLAB Function/5(HiX_PositiveY_Gradient)
  [VoltWattHiChargeGradientPU] -> MATLAB Function/6(HiX_NegativeY_Gradient)
  [VoltWattLoStartVoltagePU] -> MATLAB Function/7(LoStartX)
  [VoltWattLoStopVoltagePU] -> MATLAB Function/8(LoStopX)
  [VoltWattLoDischargeGradientPU] -> MATLAB Function/9(LoX_PositiveY_Gradient)
  [VoltWattLoChargeGradientPU] -> MATLAB Function/10(LoX_NegativeY_Gradient)
  [VoltWattStartDelay] -> MATLAB Function/11(StartDelay)
  [VoltWattStopDelay] -> MATLAB Function/12(StopDelay)
  Bus Selector4/1 -> [VoltWattHiStartVoltagePU]  "<VoltWattHiStartVoltagePU>"
  Bus Selector4/2 -> [VoltWattHiStopVoltagePU]  "<VoltWattHiStopVoltagePU>"
  Bus Selector4/3 -> [VoltWattHiDischargeGradientPU]  "<VoltWattHiDischargeGradientPU>"
  Bus Selector4/4 -> [VoltWattHiChargeGradientPU]  "<VoltWattHiChargeGradientPU>"
  Bus Selector4/5 -> [VoltWattLoStartVoltagePU]  "<VoltWattLoStartVoltagePU>"
  Bus Selector4/6 -> [VoltWattLoStopVoltagePU]  "<VoltWattLoStopVoltagePU>"
  Bus Selector4/7 -> [VoltWattLoDischargeGradientPU]  "<VoltWattLoDischargeGradientPU>"
  Bus Selector4/8 -> [VoltWattLoChargeGradientPU]  "<VoltWattLoChargeGradientPU>"
  Bus Selector4/9 -> [VoltWattStartDelay]  "<VoltWattStartDelay>"
  Bus Selector4/10 -> [VoltWattStopDelay]  "<VoltWattStopDelay>"

== system ESSLibrary/WattVarMode ==
  ActivePowerMeasPU : Inport
  WattVarOperatingParametersPU : Inport  Port=2  OutDataTypeStr=Bus: WattVarOperatingParametersPU
  Action Port : ActionPort
  Bus Selector2 : BusSelector  OutputSignals=WattVarHighStartingWattagePU,WattVarHighStoppingWattagePU,WattVarHighWattageGradientPU,WattVarLowStartingWattagePU,WattVarLowStoppingWattagePU,WattVarLowWattageGradientPU,WattVarOffsetReactivePowerPU
  Constant1 : Constant  Value=0.0  OutDataTypeStr=double  SampleTime=-1
  MATLAB Function1 : MATLAB Function  TreatAsAtomicUnit=on
  ReactivePowerOut : Outport  OutDataTypeStr=double
  wires:
  WattVarOperatingParametersPU/1 -> Bus Selector2/1
  ActivePowerMeasPU/1 -> MATLAB Function1/1(X_In)
  MATLAB Function1/1(Y_Out) -> ReactivePowerOut/1
  Constant1/1 -> MATLAB Function1/10(StopDelay), MATLAB Function1/9(StartDelay)
  Bus Selector2/4 -> MATLAB Function1/5(X_Lo_Stop)  "<WattVarLowStartingWattagePU>"
  Bus Selector2/3 -> MATLAB Function1/4(X_Lo_Start)  "<WattVarHighWattageGradientPU>"
  Bus Selector2/5 -> MATLAB Function1/6(X_Hi_Gradient)  "<WattVarLowStoppingWattagePU>"
  Bus Selector2/2 -> MATLAB Function1/3(X_Hi_Stop)  "<WattVarHighStoppingWattagePU>"
  Bus Selector2/6 -> MATLAB Function1/7(X_Lo_Gradient)  "<WattVarLowWattageGradientPU>"
  Bus Selector2/1 -> MATLAB Function1/2(X_Hi_Start)  "<WattVarHighStartingWattagePU>"
  Bus Selector2/7 -> MATLAB Function1/8(Y_Offset)  "<WattVarOffsetReactivePowerPU>"

== system ESSLibrary/ActivePowerSmoothing/MovAvgDeltaVoltCalc ==
  Enable : Inport
  Inp : Inport  Port=2
  FilterTime : Inport  Port=3
  TimeStep : Inport  Port=4
  ElseMovAvgFilter : Subsystem  TreatAsAtomicUnit=on
  If : If  IfExpression=u1 ~= 0
  IfMovAvgFilter : Subsystem  TreatAsAtomicUnit=on
  Inp1 : InportShadow  Port=2
  Switch : Switch  Criteria=u2 > Threshold
  Switch1 : Switch  Criteria=u2 > Threshold
  Out : Outport
  ErrorCode : Outport  Port=2
  wires:
  [ElseErrorCode] -> Switch1/3
  [IfErrorCode] -> Switch1/1
  [IfOut] -> Switch/1
  [ElseOut] -> Switch/3
  Switch/1 -> Out/1
  Switch1/1 -> ErrorCode/1
  IfMovAvgFilter/2(ErrorCode) -> [IfErrorCode]
  IfMovAvgFilter/1(Out) -> [IfOut]
  ElseMovAvgFilter/2(ErrorCode) -> [ElseErrorCode]
  ElseMovAvgFilter/1(Out) -> [ElseOut]
  Inp1/1 -> ElseMovAvgFilter/1(Inp)
  FilterTime/1 -> IfMovAvgFilter/2(FilterTime)
  TimeStep/1 -> IfMovAvgFilter/3(TimeStep)
  Inp/1 -> IfMovAvgFilter/1(Inp)
  If/1 -> IfMovAvgFilter/Action
  If/2 -> ElseMovAvgFilter/Action
  Enable/1 -> If/1, Switch/2, Switch1/2

== system ESSLibrary/ChargeDischargeStorageMode/Comparator ==
  note: LowerThresholdID
  note: UpperThresholdID
  note: CategoryID = 1
  Enable/Disable : Inport
  "Input " : Inport  Port=2
  UpperTrhd : Inport  Port=3
  LowerTrhd : Inport  Port=4
  HystSelection : Inport  Port=5
  AbsHyst : Inport  Port=6
  RelHyst : Inport  Port=7
  VariableIdentifier : Inport  Port=8
  Basic alarm ver2.0 : Subsystem
  CategoryID : Constant  OutDataTypeStr=int64
  Constant1 : Constant  OutDataTypeStr=int64
  Constant10 : Constant  Value=0  OutDataTypeStr=int64
  Constant11 : Constant  Value=0  OutDataTypeStr=int64
  Constant2 : Constant  Value=2  OutDataTypeStr=int64
  Gain : Gain  Gain=100
  Gain1 : Gain  Gain=10000
  Sum : Sum  Inputs=+++  OutDataTypeStr=int64
  Switch1 : Switch  Criteria=u2 ~= 0  OutDataTypeStr=int64
  Switch2 : Switch  Criteria=u2 ~= 0  OutDataTypeStr=int64
  Switch3 : Switch  Criteria=u2 ~= 0  OutDataTypeStr=int64
  Terminator1 : Terminator
  ErrorCode : Outport
  MaxLimitCrossed : Outport  Port=2
  MinLimitCrossed : Outport  Port=3
  wires:
  Basic alarm ver2.0/1(MaxLimitCrossed) -> MaxLimitCrossed/1, Switch1/2
  Constant2/1 -> Switch2/1
  CategoryID/1 -> Gain/1
  Switch1/1 -> Switch3/2, Sum/1
  Constant1/1 -> Switch1/1
  Constant11/1 -> Switch2/3
  HystSelection/1 -> Basic alarm ver2.0/5(HystSelection)
  Basic alarm ver2.0/2(MinLimitCrossed) -> MinLimitCrossed/1, Switch2/2
  Constant10/1 -> Switch3/3
  Basic alarm ver2.0/3(ErrorCode) -> Terminator1/1
  Sum/1 -> Switch3/1
  "Input "/1 -> Basic alarm ver2.0/2("Input ")
  Switch2/1 -> Switch1/3
  VariableIdentifier/1 -> Gain1/1
  AbsHyst/1 -> Basic alarm ver2.0/6(AbsHyst)
  RelHyst/1 -> Basic alarm ver2.0/7(RelHyst)
  Enable/Disable/1 -> Basic alarm ver2.0/1(Enable/disable)
  Switch3/1 -> ErrorCode/1
  UpperTrhd/1 -> Basic alarm ver2.0/3(UpperTrhd)
  LowerTrhd/1 -> Basic alarm ver2.0/4(LowerTrhd)
  Gain/1 -> Sum/2
  Gain1/1 -> Sum/3

== system ESSLibrary/Comparator/Basic alarm ver2.0 ==
  Enable/disable : Inport  OutDataTypeStr=boolean
  "Input " : Inport  Port=2
  UpperTrhd : Inport  Port=3
  LowerTrhd : Inport  Port=4
  HystSelection : Inport  Port=5  OutDataTypeStr=int32
  AbsHyst : Inport  Port=6
  RelHyst : Inport  Port=7
  Enable/disable1 : InportShadow  OutDataTypeStr=boolean
  Enabled Subsystem : Subsystem  TreatAsAtomicUnit=on
  Enabled Subsystem1 : Subsystem  TreatAsAtomicUnit=on
  If : If  IfExpression=u1 ~=0
  Switch : Switch  Criteria=u2 > Threshold
  Switch1 : Switch  Criteria=u2 > Threshold
  Switch3 : Switch  Criteria=u2 > Threshold
  MaxLimitCrossed : Outport  OutDataTypeStr=boolean
  MinLimitCrossed : Outport  Port=2  OutDataTypeStr=boolean
  ErrorCode : Outport  Port=3  OutDataTypeStr=int64
  wires:
  Enable/disable/1 -> If/1
  If/2 -> Enabled Subsystem/Action
  If/1 -> Enabled Subsystem1/Action
  Enabled Subsystem1/3(ErrorCode) -> [If_Errorcode]
  Enabled Subsystem/2(ErrorCode) -> [Else_Errorcode]
  Enabled Subsystem/1("MaxLimitCrossed ") -> [Else_MaxLimitCrossed]
  [If_MaxLimitCrossed] -> Switch/1
  [If_Errorcode] -> Switch3/1
  [Else_Errorcode] -> Switch3/3
  Enabled Subsystem1/1(MaxLimitCrossed) -> [If_MaxLimitCrossed]
  Switch/1 -> MaxLimitCrossed/1
  [Else_MaxLimitCrossed] -> Switch/3
  Enable/disable1/1 -> Switch3/2, Switch1/2, Switch/2
  "Input "/1 -> Enabled Subsystem1/1("Input ")
  UpperTrhd/1 -> Enabled Subsystem1/2(UpperTrhd)
  LowerTrhd/1 -> Enabled Subsystem1/3(LowerTrhd)
  AbsHyst/1 -> Enabled Subsystem1/5(AbsHyst)
  RelHyst/1 -> Enabled Subsystem1/6(RelHyst)
  HystSelection/1 -> Enabled Subsystem1/4(HystSelection)
  Enabled Subsystem1/2(MinLimitCrossed) -> [If_MinLimitCrossed]
  Enabled Subsystem/3(MinLimitCrossed) -> [Else_MinLimitCrossed]
  [If_MinLimitCrossed] -> Switch1/1
  [Else_MinLimitCrossed] -> Switch1/3
  Switch1/1 -> MinLimitCrossed/1
  Switch3/1 -> ErrorCode/1

== system ESSLibrary/CoordinatedChDischMode/EnabledCoordinatedChDischMode ==
  ActvPowMeasPU : Inport
  SoC : Inport  Port=2
  TimeStep : Inport  Port=3
  BattCapacity : Inport  Port=4
  TargetSOC : Inport  Port=5
  MinChargeDuration : Inport  Port=6
  ActivePowerRampUpRate : Inport  Port=7
  ActivePowerRampDownRate : Inport  Port=8
  Abs : Abs
  ActvPowMeasPU1 : InportShadow
  ActvPowMeasPU2 : InportShadow
  CrdChDischActivePowerEvaluator : MATLAB Function  TreatAsAtomicUnit=on
  Gain1 : Gain  Gain=-1
  GreaterThan2 : RelationalOperator  Operator=>  OutDataTypeStr=boolean  RndMeth=Simplest
  Scope : Scope  NumInputPorts=3
  Scope3 : Scope  NumInputPorts=2
  Scope7 : Scope  NumInputPorts=2
  Switch7 : Switch
  Terminator : Terminator
  TimeStep1 : InportShadow  Port=3
  TimeTrigger : MATLAB Function  TreatAsAtomicUnit=on
  ActivePowerOut : Outport
  FailOperationErrorCode : Outport  Port=2
  wires:
  CrdChDischActivePowerEvaluator/1(Pout) -> Scope7/1, [Preq]
  TimeStep1/1 -> TimeTrigger/4(TimeStep)
  ActvPowMeasPU1/1 -> Abs/1
  CrdChDischActivePowerEvaluator/2(Tout) -> [Treq], Scope7/2
  [Treq] -> Scope/2, TimeTrigger/2(TimeRequired)
  TimeStep/1 -> CrdChDischActivePowerEvaluator/5(TimeStep)
  ActivePowerRampDownRate/1 -> CrdChDischActivePowerEvaluator/8(CrdChDischModeRampDown)
  ActivePowerRampUpRate/1 -> CrdChDischActivePowerEvaluator/7(CrdChDischModeRampUp)
  MinChargeDuration/1 -> CrdChDischActivePowerEvaluator/4(MaxChOrDischDuration)
  TargetSOC/1 -> [TargetSoC], CrdChDischActivePowerEvaluator/3(SoCTarget)
  SoC/1 -> CrdChDischActivePowerEvaluator/2(SoCMeas), [SoC], Scope3/2
  BattCapacity/1 -> CrdChDischActivePowerEvaluator/6(BattCapacity)
  [Preq] -> TimeTrigger/1(ActivePowerRequired)
  Abs/1 -> Scope/3, TimeTrigger/3(ActivePowerMeas)
  [SoC] -> GreaterThan2/2
  [TargetSoC] -> GreaterThan2/1
  GreaterThan2/1 -> Switch7/2
  ActvPowMeasPU/1 -> Switch7/3
  Switch7/1 -> Scope3/1, CrdChDischActivePowerEvaluator/1(ActivePowerMeas)
  ActvPowMeasPU2/1 -> Gain1/1
  Gain1/1 -> Switch7/1
  TimeTrigger/1(flag) -> Terminator/1
  TimeTrigger/2(ActivePowerOut) -> ActivePowerOut/1
  CrdChDischActivePowerEvaluator/3(ErrorCode) -> FailOperationErrorCode/1

== system ESSLibrary/Disconnected/If Action Subsystem ==
  Action Port : ActionPort  ActionPortLabel=else
  Constant1 : Constant  Value=0  OutDataTypeStr=int64  SampleTime=-1
  Constant2 : Constant  Value=0  OutDataTypeStr=boolean  SampleTime=-1
  Constant6 : Constant  Value=0  OutDataTypeStr=double  SampleTime=-1
  ActivePowerOut : Outport  OutDataTypeStr=double
  ReactivePowerOut : Outport  Port=2  OutDataTypeStr=double
  OpenCmd : Outport  Port=3  OutDataTypeStr=boolean
  CloseCmd : Outport  Port=4  OutDataTypeStr=boolean
  ErrorCode : Outport  Port=5  OutDataTypeStr=int64
  wires:
  Constant6/1 -> ReactivePowerOut/1, ActivePowerOut/1
  Constant2/1 -> CloseCmd/1, OpenCmd/1
  Constant1/1 -> ErrorCode/1

== system ESSLibrary/Disconnected/IfActionSubsystem ==
  CBStatus : Inport  OutDataTypeStr=int8
  ZeroActivePowerFlow : Inport  Port=2  OutDataTypeStr=boolean
  ZeroReactivePowerFlow : Inport  Port=3  OutDataTypeStr=boolean
  BreakerCmdTime : Inport  Port=4
  OpenTimeOut : Inport  Port=5
  ResetDisconnected : Inport  Port=6
  LogicalBlockID : Inport  Port=7  OutDataTypeStr=int64
  Action Port : ActionPort  ActionPortLabel=if(u1 ~= 0)
  Constant26 : Constant  Value=0  OutDataTypeStr=int64
  Constant27 : Constant  Value=0  OutDataTypeStr=int64
  DisconnectedMode : MATLAB Function  TreatAsAtomicUnit=on
  Equal2 : RelationalOperator  Operator=>  OutDataTypeStr=boolean  RndMeth=Simplest
  Gain : Gain  Gain=1000000
  Sum2 : Sum  OutDataTypeStr=int64
  Switch1 : Switch  Criteria=u2 > Threshold
  ActivePowerOut : Outport
  ReactivePowerOut : Outport  Port=2
  OpenCmd : Outport  Port=3
  CloseCmd : Outport  Port=4
  ErrorCode : Outport  Port=5  OutDataTypeStr=int64
  wires:
  BreakerCmdTime/1 -> DisconnectedMode/4(BreakerCmdTime)
  ZeroReactivePowerFlow/1 -> DisconnectedMode/3(ZeroReactivePowerFlow)
  ZeroActivePowerFlow/1 -> DisconnectedMode/2(ZeroActivePowerFlow)
  CBStatus/1 -> DisconnectedMode/1(CBStatus)
  DisconnectedMode/3(OpenCmd) -> OpenCmd/1
  DisconnectedMode/4(CloseCmd) -> CloseCmd/1
  Equal2/1 -> Switch1/2
  Switch1/1 -> ErrorCode/1
  Constant27/1 -> Switch1/3
  LogicalBlockID/1 -> Gain/1
  Gain/1 -> Sum2/2
  Constant26/1 -> Equal2/2
  DisconnectedMode/5(ErrorCode) -> Sum2/1, Equal2/1
  Sum2/1 -> Switch1/1
  DisconnectedMode/1(ActivePowerOut) -> ActivePowerOut/1
  DisconnectedMode/2(ReactivePowerOut) -> ReactivePowerOut/1
  OpenTimeOut/1 -> DisconnectedMode/5(OpenTimeOut)
  ResetDisconnected/1 -> DisconnectedMode/6(ResetDisconnected)

== system ESSLibrary/Dispatch/ElseActionSubsystem ==
  Action Port : ActionPort
  Constant1 : Constant  Value=0  OutDataTypeStr=double  SampleTime=-1
  Constant2 : Constant  Value=0  OutDataTypeStr=boolean  SampleTime=-1
  Constant3 : Constant  Value=0  OutDataTypeStr=int8  SampleTime=-1
  Constant4 : Constant  Value=0  OutDataTypeStr=int32  SampleTime=-1
  OperationMode : Outport  OutDataTypeStr=int8
  ActivePowerMode : Outport  Port=2  OutDataTypeStr=int8
  ReactivePowerMode : Outport  Port=3  OutDataTypeStr=int8
  ActivePowerOut : Outport  Port=4  OutDataTypeStr=double
  ReactvPowerOut : Outport  Port=5  OutDataTypeStr=double
  OpenCmd : Outport  Port=6  OutDataTypeStr=boolean
  CloseCmd : Outport  Port=7  OutDataTypeStr=boolean
  ErrorCode : Outport  Port=8  OutDataTypeStr=int32
  wires:
  Constant1/1 -> ReactvPowerOut/1, ActivePowerOut/1
  Constant2/1 -> CloseCmd/1, OpenCmd/1
  Constant3/1 -> ReactivePowerMode/1, ActivePowerMode/1, OperationMode/1
  Constant4/1 -> ErrorCode/1
